simulink model "k1vispr2"  (Simulink 8.5)
settings: Solver=ode45  StartTime=0.0  StopTime=10.0  RelTol=1e-3
undefined symbols (not defined in the file): AC, SIXOSEM_F_WD_AC_MASTER
libraries: cdsFiltCtrl x19, cdsEpicsOut x13, cdsFilt x12, cdsTP x12, cdsRms x6, cdsMuxMatrix x3, cdsFunctionCall x1, cdsEpicsIn x1, SIXOSEM_F_STAGE_MASTER x1, cdsEpicsBinIn x1, cdsEpicsMomentary x1, cdsAdcx0 x1
(part 1 of 5)
settings Model: Creator=controls  LastModifiedBy=controls
settings OptimizationCC: InitFltsAndDblsToZero=on
settings DebuggingCC: SolverPrmCheckMsg=warning  FcnCallInpInsideContextMsg=UseLocalSettings  StrictBusMsg=Warning

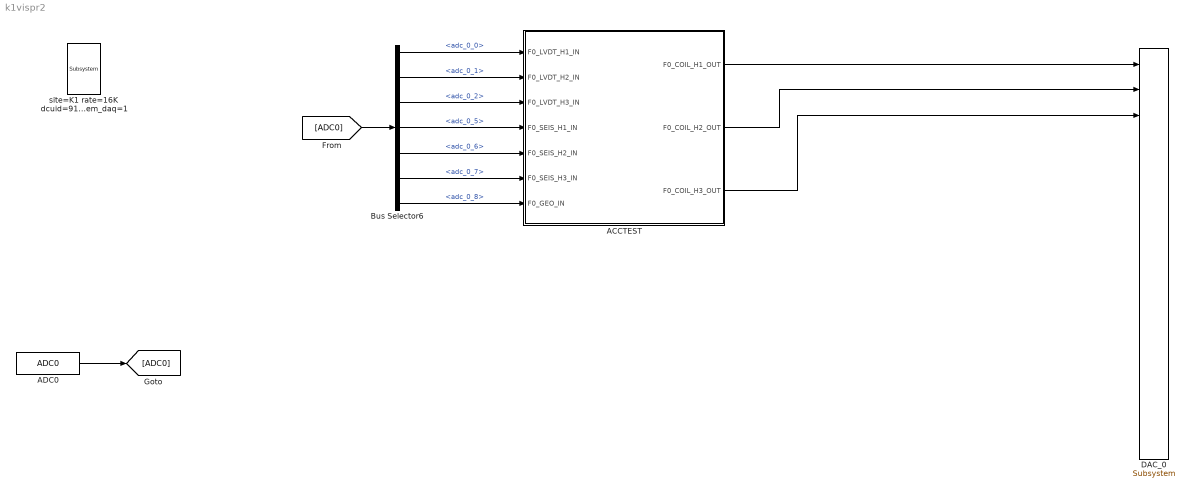
== system k1vispr2 ==
  ACCTEST : Subsystem
  ADC0 : cdsAdcx0/ADC0  Tag=cdsAdc  Description=|
      | type-GSC_16AI64SSA
      | card_num=0
      settings: AttributesFormatString=%<Description>\n%<Tag>
  Bus Selector6 : BusSelector  Description=ADC Selector  OutputSignals=adc_0_0,adc_0_1,adc_0_2,adc_0_5,adc_0_6,adc_0_7,adc_0_8
      settings: AttributesFormatString=%<Description>
  DAC_0 : dac/Subsystem  Description=|
      | type=GSC_16AO16,
      | card_num=0
      settings: AttributesFormatString=%<Description>
  site=K1 rate=16K dcuid=91 host=k1pr2 specific_cpu=3 adcSlave=1 shmem_daq=1 : cdsParameters/Subsystem  Tag=cdsParameters  Description=|
      | Purpose:                                                                                                                                                                                                                                
      | Provide system parameters to the FE code generator to properly configure the generated EPICS names, rep rate of the FE controller, and the Data Acquisition node ID for proper storage of data from this FE controller.                 
      |                                                                                                                                                                                                                                         
      | Useage:                                                                                                                                                                                                                                 
      | The part NAME field is used to identify the FE parameters. It must be of the form:                                                                                                                                                      
      | site=                                                                                                                                                                                                                                   
      | rate=                                                                                                                                                                                                                                   
      | dcuid=                                                                                                                                                                                                                                  
      |                                                                                                                                                                                                                                         
      | Where:                                                                                                                                                                                                                                  
      | site= argument may be H1, H2, L1, M1, G1, either as a single argument or multiple, for example site=H1,H2. These are the only names allowed. These will become the first two characters of all EPICS and signal names (for example G1:).
      |                                                                                                                                                                                                                                         
      | rate= may be 2K, 16K, 32K, or 64K                                                                                                                                                                                                       
      |                                                                                                                                                                                                                                         
      | dcuid= is site specific ie it must be unique at each site.
      settings: AttributesFormatString=%<Tag>
  wires:
  Bus Selector6/1 -> ACCTEST/1(F0_LVDT_H1_IN)  "<adc_0_0>"
  ADC0/1 -> [ADC0]
  [ADC0] -> Bus Selector6/1
  ACCTEST/1(F0_COIL_H1_OUT) -> DAC_0/1
  ACCTEST/2(F0_COIL_H2_OUT) -> DAC_0/2
  ACCTEST/3(F0_COIL_H3_OUT) -> DAC_0/3
  Bus Selector6/2 -> ACCTEST/2(F0_LVDT_H2_IN)  "<adc_0_1>"
  Bus Selector6/3 -> ACCTEST/3(F0_LVDT_H3_IN)  "<adc_0_2>"
  Bus Selector6/4 -> ACCTEST/4(F0_SEIS_H1_IN)  "<adc_0_5>"
  Bus Selector6/5 -> ACCTEST/5(F0_SEIS_H2_IN)  "<adc_0_6>"
  Bus Selector6/6 -> ACCTEST/6(F0_SEIS_H3_IN)  "<adc_0_7>"
  Bus Selector6/7 -> ACCTEST/7(F0_GEO_IN)  "<adc_0_8>"

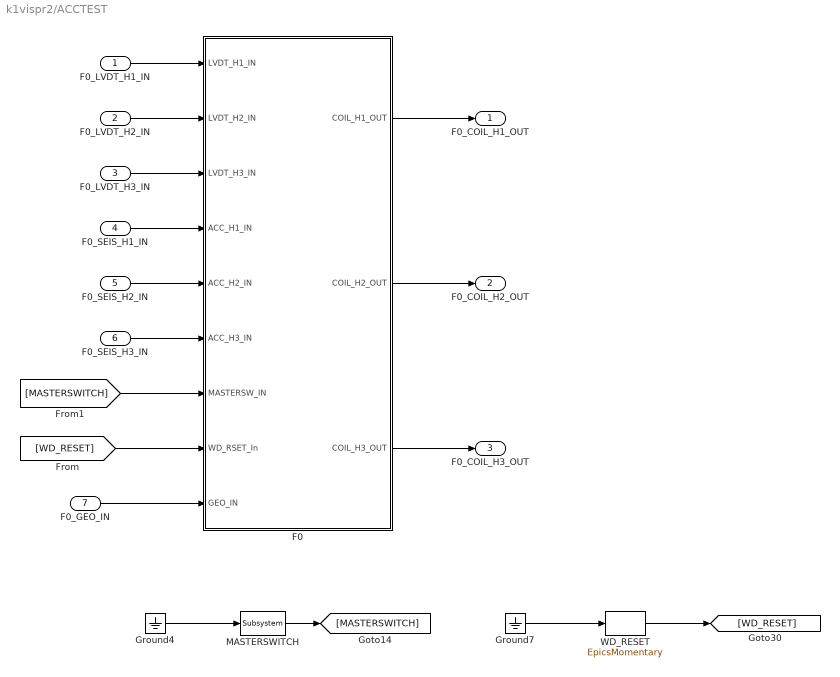
== system k1vispr2/ACCTEST ==
  F0_LVDT_H1_IN : Inport
  F0_LVDT_H2_IN : Inport  Port=2
  F0_LVDT_H3_IN : Inport  Port=3
  F0_SEIS_H1_IN : Inport  Port=4
  F0_SEIS_H2_IN : Inport  Port=5
  F0_SEIS_H3_IN : Inport  Port=6
  F0_GEO_IN : Inport  Port=7
  F0 : Subsystem
  Ground4 : Ground
  Ground7 : Ground
  MASTERSWITCH : cdsEpicsBinIn/Subsystem  Tag=cdsEpicsBinIn  Description=|
      | Purpose:                                                                            
      | Create an EPICS binary (0 or 1) input channel to the FE realtime controls.          
      |                                                                                     
      | Operation:                                                                          
      | Outputs value from an EPICS ai record. Value is binary input (bi Epics record type).
      |                                                                                     
      | Usage:                                                                              
      | Name the part with the desired EPICS channel name.
      settings: AttributesFormatString=%<Tag>
  WD_RESET : cdsEpicsMomentary/EpicsMomentary  Tag=cdsEpicsMomentary
      settings: AttributesFormatString=%<Tag>
  F0_COIL_H1_OUT : Outport
  F0_COIL_H2_OUT : Outport  Port=2
  F0_COIL_H3_OUT : Outport  Port=3
  wires:
  F0/1(COIL_H1_OUT) -> F0_COIL_H1_OUT/1
  F0/2(COIL_H2_OUT) -> F0_COIL_H2_OUT/1
  F0/3(COIL_H3_OUT) -> F0_COIL_H3_OUT/1
  F0_LVDT_H1_IN/1 -> F0/1(LVDT_H1_IN)
  F0_LVDT_H2_IN/1 -> F0/2(LVDT_H2_IN)
  F0_LVDT_H3_IN/1 -> F0/3(LVDT_H3_IN)
  F0_SEIS_H1_IN/1 -> F0/4(ACC_H1_IN)
  F0_SEIS_H2_IN/1 -> F0/5(ACC_H2_IN)
  F0_SEIS_H3_IN/1 -> F0/6(ACC_H3_IN)
  [MASTERSWITCH] -> F0/7(MASTERSW_IN)
  MASTERSWITCH/1 -> [MASTERSWITCH]
  Ground4/1 -> MASTERSWITCH/1
  Ground7/1 -> WD_RESET/1
  WD_RESET/1 -> [WD_RESET]
  [WD_RESET] -> F0/8(WD_RSET_In)
  F0_GEO_IN/1 -> F0/9(GEO_IN)

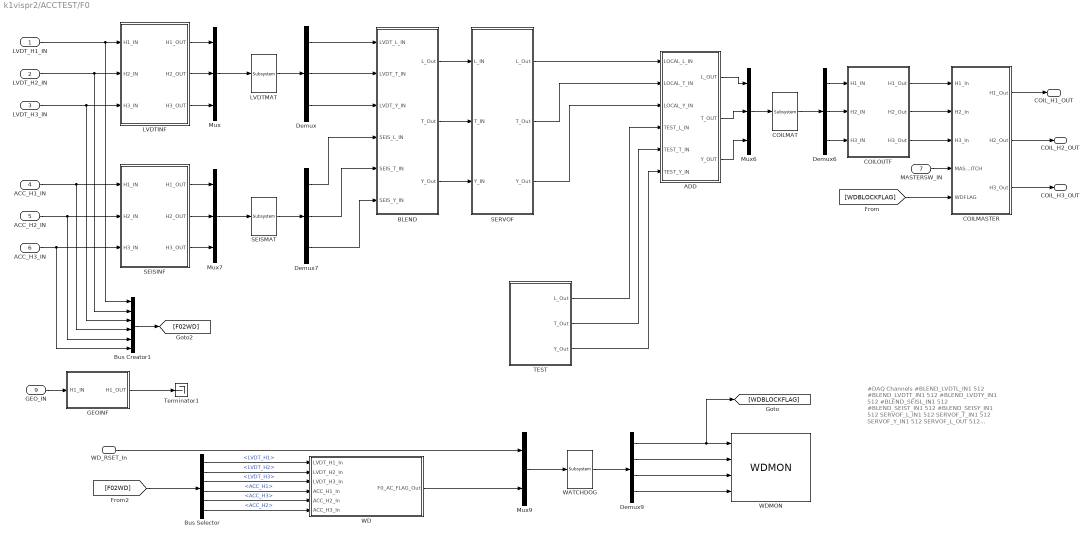
== system k1vispr2/ACCTEST/F0 ==
  note: #DAQ Channels
      |
      | #BLEND_LVDTL_IN1 512
      | #BLEND_LVDTT_IN1 512
      | #BLEND_LVDTY_IN1 512
      | #BLEND_SEISL_IN1 512
      | #BLEND_SEIST_IN1 512
      | #BLEND_SEISY_IN1 512
      | SERVOF_L_IN1 512
      | SERVOF_T_IN1 512
      | SERVOF_Y_IN1 512
      | SERVOF_L_OUT 512
      | SERVOF_T_OUT 512
      | SERVOF_Y_OUT 512
      | ADD_L_OUT 512
      | ADD_T_OUT 512
      | ADD_Y_OUT 512
      | #COILMASTER_H1_MON 512
      | #COILMASTER_H2_MON 512
      | #COILMASTER_H3_MON 512
  LVDT_H1_IN : Inport
  LVDT_H2_IN : Inport  Port=2
  LVDT_H3_IN : Inport  Port=3
  ACC_H1_IN : Inport  Port=4
  ACC_H2_IN : Inport  Port=5
  ACC_H3_IN : Inport  Port=6
  MASTERSW_IN : Inport  Port=7
  WD_RSET_In : Inport  Port=8
  GEO_IN : Inport  Port=9
  ADD : Subsystem
  BLEND : Subsystem
  Bus Creator1 : BusCreator  Inputs='LVDT_H1','LVDT_H2','LVDT_H3','ACC_H1','ACC_H2','ACC_H3'
  Bus Selector : BusSelector  OutputSignals=LVDT_H1,LVDT_H2,LVDT_H3,ACC_H1,ACC_H3,ACC_H2
  COILMASTER : Subsystem
  COILMAT : cdsMuxMatrix/Subsystem  Tag=cdsMuxMatrix  Description=|
      | ADL=SUS_INMATRIX.adl                                                                
      | SCRIPT=generate_KisselButton.py 4 5 #CHANNEL# > #TARGET_DIR#/#FULL_PART_NAME#_KB.adl
      settings: AttributesFormatString=%<Tag>
  COILOUTF : Subsystem
  Demux : Demux  Outputs=3
  Demux6 : Demux  Outputs=3
  Demux7 : Demux  Outputs=3
  Demux9 : Demux
  GEOINF : Subsystem
  LVDTINF : Subsystem
  LVDTMAT : cdsMuxMatrix/Subsystem  Tag=cdsMuxMatrix  Description=|
      | ADL=SUS_INMATRIX.adl                                                                
      | SCRIPT=generate_KisselButton.py 4 5 #CHANNEL# > #TARGET_DIR#/#FULL_PART_NAME#_KB.adl
      settings: AttributesFormatString=%<Tag>
  Mux : Mux  Inputs=3
  Mux6 : Mux  Inputs=3
  Mux7 : Mux  Inputs=3
  Mux9 : Mux  Inputs=2
  SEISINF : Subsystem
  SEISMAT : cdsMuxMatrix/Subsystem  Tag=cdsMuxMatrix  Description=|
      | ADL=SUS_INMATRIX.adl                                                                
      | SCRIPT=generate_KisselButton.py 4 5 #CHANNEL# > #TARGET_DIR#/#FULL_PART_NAME#_KB.adl
      settings: AttributesFormatString=%<Tag>
  SERVOF : Subsystem
  TEST : Subsystem
  Terminator1 : Terminator
  WATCHDOG : cdsFunctionCall/Subsystem  Tag=cdsFunctionCall  Description=inline OSEMWATCHDOG /opt/rtcds/userapps/release/vis/common/src/WATCHDOG.c
      settings: AttributesFormatString=%<Tag>\n%<Description>
  WD : Subsystem  AncestorBlock=SIXOSEM_F_STAGE_MASTER/SIXOSEM_F_STAGE_MASTER/WD
  WDMON : SIXOSEM_F_STAGE_MASTER/SIXOSEM_F_STAGE_MASTER/WDMON
  COIL_H1_OUT : Outport
  COIL_H2_OUT : Outport  Port=2
  COIL_H3_OUT : Outport  Port=3
  wires:
  LVDTINF/1(H1_OUT) -> Mux/1
  LVDTINF/2(H2_OUT) -> Mux/2
  LVDTINF/3(H3_OUT) -> Mux/3
  Mux/1 -> LVDTMAT/1
  LVDTMAT/1 -> Demux/1
  Mux7/1 -> SEISMAT/1
  SEISINF/1(H1_OUT) -> Mux7/1
  SEISINF/3(H3_OUT) -> Mux7/3
  SEISINF/2(H2_OUT) -> Mux7/2
  SEISMAT/1 -> Demux7/1
  Demux/1 -> BLEND/1(LVDT_L_IN)
  Demux/2 -> BLEND/2(LVDT_T_IN)
  Demux/3 -> BLEND/3(LVDT_Y_IN)
  Demux7/1 -> BLEND/4(SEIS_L_IN)
  Demux7/2 -> BLEND/5(SEIS_T_IN)
  Demux7/3 -> BLEND/6(SEIS_Y_IN)
  BLEND/1(L_Out) -> SERVOF/1(L_IN)
  BLEND/2(T_Out) -> SERVOF/2(T_IN)
  BLEND/3(Y_Out) -> SERVOF/3(Y_IN)
  SERVOF/1(L_Out) -> ADD/1(LOCAL_L_IN)
  SERVOF/2(T_Out) -> ADD/2(LOCAL_T_IN)
  SERVOF/3(Y_Out) -> ADD/3(LOCAL_Y_IN)
  ADD/1(L_OUT) -> Mux6/1
  ADD/2(T_OUT) -> Mux6/2
  ADD/3(Y_OUT) -> Mux6/3
  Mux6/1 -> COILMAT/1
  COILMAT/1 -> Demux6/1
  Demux6/1 -> COILOUTF/1(H1_IN)
  Demux6/2 -> COILOUTF/2(H2_IN)
  Demux6/3 -> COILOUTF/3(H3_IN)
  COILMASTER/1(H1_Out) -> COIL_H1_OUT/1
  COILMASTER/2(H2_Out) -> COIL_H2_OUT/1
  COILMASTER/3(H3_Out) -> COIL_H3_OUT/1
  TEST/1(L_Out) -> ADD/4(TEST_L_IN)
  TEST/2(T_Out) -> ADD/5(TEST_T_IN)
  TEST/3(Y_Out) -> ADD/6(TEST_Y_IN)
  COILOUTF/1(H1_Out) -> COILMASTER/1(H1_In)
  COILOUTF/2(H2_Out) -> COILMASTER/2(H2_In)
  COILOUTF/3(H3_Out) -> COILMASTER/3(H3_In)
  MASTERSW_IN/1 -> COILMASTER/4(MASTERSWITCH)
  WD_RSET_In/1 -> Mux9/1
  WD/1(F0_AC_FLAG_Out) -> Mux9/2
  [F02WD] -> Bus Selector/1
  Bus Selector/1 -> WD/1(LVDT_H1_In)  "<LVDT_H1>"
  Bus Selector/2 -> WD/2(LVDT_H2_In)  "<LVDT_H2>"
  Bus Selector/3 -> WD/3(LVDT_H3_In)  "<LVDT_H3>"
  Bus Selector/4 -> WD/4(ACC_H1_In)  "<ACC_H1>"
  Bus Selector/5 -> WD/5(ACC_H2_In)  "<ACC_H3>"
  Bus Selector/6 -> WD/6(ACC_H3_In)  "<ACC_H2>"
  Demux9/1 -> [WDBLOCKFLAG], WDMON/1
  Demux9/2 -> WDMON/2
  Demux9/3 -> WDMON/3
  Demux9/4 -> WDMON/4
  Mux9/1 -> WATCHDOG/1
  WATCHDOG/1 -> Demux9/1
  LVDT_H1_IN/1 -> Bus Creator1/1, LVDTINF/1(H1_IN)
  LVDT_H2_IN/1 -> Bus Creator1/2, LVDTINF/2(H2_IN)
  LVDT_H3_IN/1 -> Bus Creator1/3, LVDTINF/3(H3_IN)
  ACC_H1_IN/1 -> Bus Creator1/4, SEISINF/1(H1_IN)
  ACC_H2_IN/1 -> Bus Creator1/5, SEISINF/2(H2_IN)
  ACC_H3_IN/1 -> Bus Creator1/6, SEISINF/3(H3_IN)
  Bus Creator1/1 -> [F02WD]
  [WDBLOCKFLAG] -> COILMASTER/5(WDFLAG)
  GEO_IN/1 -> GEOINF/1(H1_IN)
  GEOINF/1(H1_OUT) -> Terminator1/1

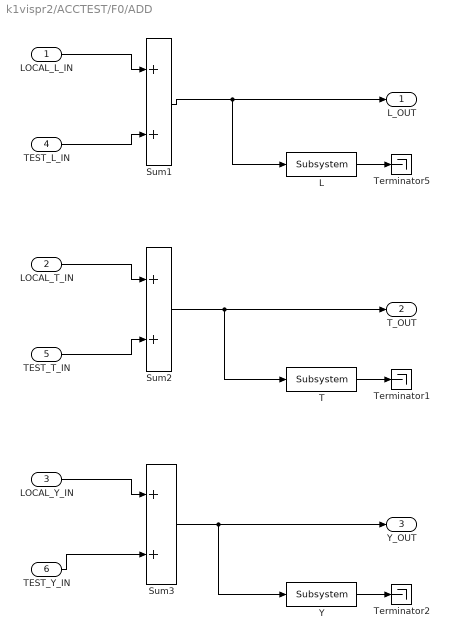
== system k1vispr2/ACCTEST/F0/ADD ==
  LOCAL_L_IN : Inport
  LOCAL_T_IN : Inport  Port=2
  LOCAL_Y_IN : Inport  Port=3
  TEST_L_IN : Inport  Port=4
  TEST_T_IN : Inport  Port=5
  TEST_Y_IN : Inport  Port=6
  L : cdsFilt/Subsystem  Tag=cdsFilt  Description=|
      | Purpose:                                                                                                                                                                                                                                  
      | Standard CDS IIR filter module.                                                                                                                                                                                                           
      |                                                                                                                                                                                                                                           
      | Operation:                                                                                                                                                                                                                                
      | Consists of 10 second order section IIR filters, plus a ramped gain stage. In FE code, also provides pre-defined test points and excitation channel inputs. The filter coefficients are defined in the LIGO system using the 'foton' tool.
      |                                                                                                                                                                                                                                           
      | Usage:                                                                                                                                                                                                                                    
      | Name the part with the desired filter module name.
      settings: AttributesFormatString=%<Tag>
  Sum1 : Sum
  Sum2 : Sum
  Sum3 : Sum
  T : cdsFilt/Subsystem  Tag=cdsFilt  Description=|
      | Purpose:                                                                                                                                                                                                                                  
      | Standard CDS IIR filter module.                                                                                                                                                                                                           
      |                                                                                                                                                                                                                                           
      | Operation:                                                                                                                                                                                                                                
      | Consists of 10 second order section IIR filters, plus a ramped gain stage. In FE code, also provides pre-defined test points and excitation channel inputs. The filter coefficients are defined in the LIGO system using the 'foton' tool.
      |                                                                                                                                                                                                                                           
      | Usage:                                                                                                                                                                                                                                    
      | Name the part with the desired filter module name.
      settings: AttributesFormatString=%<Tag>
  Terminator1 : Terminator
  Terminator2 : Terminator
  Terminator5 : Terminator
  Y : cdsFilt/Subsystem  Tag=cdsFilt  Description=|
      | Purpose:                                                                                                                                                                                                                                  
      | Standard CDS IIR filter module.                                                                                                                                                                                                           
      |                                                                                                                                                                                                                                           
      | Operation:                                                                                                                                                                                                                                
      | Consists of 10 second order section IIR filters, plus a ramped gain stage. In FE code, also provides pre-defined test points and excitation channel inputs. The filter coefficients are defined in the LIGO system using the 'foton' tool.
      |                                                                                                                                                                                                                                           
      | Usage:                                                                                                                                                                                                                                    
      | Name the part with the desired filter module name.
      settings: AttributesFormatString=%<Tag>
  L_OUT : Outport
  T_OUT : Outport  Port=2
  Y_OUT : Outport  Port=3
  wires:
  LOCAL_L_IN/1 -> Sum1/1
  LOCAL_Y_IN/1 -> Sum3/1
  LOCAL_T_IN/1 -> Sum2/1
  Sum1/1 -> L/1, L_OUT/1
  Sum2/1 -> T/1, T_OUT/1
  Sum3/1 -> Y/1, Y_OUT/1
  TEST_L_IN/1 -> Sum1/2
  TEST_T_IN/1 -> Sum2/2
  TEST_Y_IN/1 -> Sum3/2
  L/1 -> Terminator5/1
  T/1 -> Terminator1/1
  Y/1 -> Terminator2/1
